simulink model "takeoff_real23B"  (R2023b)
settings: Solver=ode4  StartTime=0.0  StopTime=150  FixedStep=0.001  RelTol=1e-3
values from neighbouring files (symbols this model uses):
  a0 = 340.294    [basedata.m]    (also in basedata.mat; control_design.mat; landing_init.m; landing_plan.mat)
  b_ref = 2.0    (= 2)    [basedata.m]    (also in basedata.mat; control_design.mat; landing_init.m; landing_plan.mat)
  c_gear = [0.8e4, 1.4e4, 1.4e4]    [basedata.m]    (also in basedata.mat = [8000 14000 14000]; control_design.mat = [8000 14000 14000]; landing_init.m; landing_plan.mat = [8000 14000 14000])
  c_lat = [1.4e4, 2.2e4, 2.2e4]    [basedata.m]    (also in basedata.mat = [14000 22000 22000]; control_design.mat = [14000 22000 22000]; landing_init.m; landing_plan.mat = [14000 22000 22000])
  c_ref = 0.9    [basedata.m]    (also in basedata.mat; control_design.mat; landing_init.m; landing_plan.mat)
  c_roll = [0.020, 0.018, 0.018]    [basedata.m]    (also in basedata.mat = [0.02 0.018 0.018]; control_design.mat = [0.02 0.018 0.018]; landing_init.m; landing_plan.mat = [0.02 0.018 0.018])
  CD0 = 0.045    [basedata.m]    (also in basedata.mat; canshujisuan.m; control_design.mat; landing_init.m)
  CL0 = 0.083    [basedata.m]    (also in basedata.mat; control_design.mat; landing_init.m; landing_plan.mat)
  CLa = 3.80    (= 3.8)    [basedata.m]    (also in basedata.mat; canshujisuan.m = 2.5; control_design.mat; landing_init.m)
  Clb = -0.08    [basedata.m]    (also in basedata.mat; control_design.mat; landing_init.m; landing_plan.mat)
  Clda = -0.20    (= -0.2)    [basedata.m]    (also in basedata.mat; control_design.mat; landing_init.m; landing_plan.mat)
  CLde = 0.28    [basedata.m]    (also in basedata.mat; control_design.mat; landing_init.m; landing_plan.mat)
  Clp = -0.70    (= -0.7)    [basedata.m]    (also in basedata.mat; control_design.mat; landing_init.m; landing_plan.mat)
  CLq = 4.50    (= 4.5)    [basedata.m]    (also in basedata.mat; canshujisuan.m = 3; control_design.mat; landing_init.m)
  Clr = 0.08    [basedata.m]    (also in basedata.mat; control_design.mat; landing_init.m; landing_plan.mat)
  Cm0 = 0.060    (= 0.06)    [basedata.m]    (also in basedata.mat; control_design.mat; landing_init.m; landing_plan.mat)
  Cma = -0.80    (= -0.8)    [basedata.m]    (also in basedata.mat; control_design.mat; landing_init.m; landing_plan.mat)
  Cmde = -0.90    (= -0.9)    [basedata.m]    (also in basedata.mat; control_design.mat; landing_init.m; landing_plan.mat)
  Cmq = -18.0    (= -18)    [basedata.m]    (also in basedata.mat; control_design.mat; landing_init.m; landing_plan.mat)
  Cnb = 0.25    [basedata.m]    (also in basedata.mat; control_design.mat; landing_init.m; landing_plan.mat)
  Cndr = -0.15    [basedata.m]    (also in basedata.mat; control_design.mat; landing_init.m; landing_plan.mat)
  Cnp = -0.04    [basedata.m]    (also in basedata.mat; control_design.mat; landing_init.m; landing_plan.mat)
  Cnr = -0.45    [basedata.m]    (also in basedata.mat; control_design.mat; landing_init.m; landing_plan.mat)
  CSb = -0.70    (= -0.7)    [basedata.m]    (also in basedata.mat; control_design.mat; landing_init.m; landing_plan.mat)
  CSdr = 0.18    [basedata.m]    (also in basedata.mat; control_design.mat; landing_init.m; landing_plan.mat)
  CSr = 0.12    [basedata.m]    (also in basedata.mat; control_design.mat; landing_init.m; landing_plan.mat)
  D = 0.5 * rho0 * V^2 * S_ref * CD_current    [canshujisuan.m]
  D0 = 1400    [basedata.m]    (also in basedata.mat; control_design.mat = 800; landing.m; landing_init.m)
  da_max = 25    [basedata.m]    (also in basedata.mat; control_design.mat; landing_init.m; landing_plan.mat)
  da_min = -da_max    (= -25)    [basedata.m]    (also in basedata.mat; control_design.mat; landing_init.m; landing_plan.mat)
  de_max = 25    [basedata.m]    (also in basedata.mat; control_design.mat; landing_init.m; landing_plan.mat)
  de_min = -de_max    (= -25)    [basedata.m]    (also in basedata.mat; control_design.mat; landing_init.m; landing_plan.mat)
  DH = pi / 180    (= 0.0174532925199)    [basedata.m]    (also in basedata.mat; control_design.mat; landing_init.m; landing_plan.mat)
  dr_max = 25    [basedata.m]    (also in basedata.mat; control_design.mat; landing_init.m; landing_plan.mat)
  dr_min = -dr_max    (= -25)    [basedata.m]    (also in basedata.mat; control_design.mat; landing_init.m; landing_plan.mat)
  g = 9.80665    [basedata.m]    (also in basedata.mat; canshujisuan.m; control_design.mat; landing_init.m)
  gamma1 = -0.125844364415    [basedata.mat]    (also in landing_trajectory.m = asin(max(min(gamma1_arg, 1), -1)); landingplan.mat)
  gamma2 = -0.0261780104712    [basedata.mat]    (also in landing_trajectory.m = -0.0261799387799; landingplan.mat = 0.0261780104712)
  ground_z = 0.0    (= 0)    [basedata.m]    (also in basedata.mat; control_design.mat; landing_init.m; landing_plan.mat)
  HD = 180 / pi    (= 57.2957795131)    [basedata.m]    (also in basedata.mat; control_design.mat; landing_init.m; landing_plan.mat)
  I = [ Ixx, -Ixy, -Ixz ... (first row only)    [basedata.m]    (also in basedata.mat = [120  0  0; 0  480  0; 0  0  520]; control_design.mat = [120  0  0; 0  480  0; 0  0  520]; landing_init.m; landing_plan.mat = [120  0  0; 0  480  0; 0  0  520])
  K = 0.12    [basedata.m]    (also in basedata.mat; canshujisuan.m = 0.08; control_design.mat; landing_init.m)
  K_alpha = 7.5375    [basedata.mat]    (also in control_design.m = (((wd_pitch^2)-a24))/(2*kesi_pitch*wd_pitch); control_design.mat; controller.m = 5; landingplan.mat)
  k_gear = [1.0e5, 3.0e5, 3.0e5]    [basedata.m]    (also in basedata.mat = [100000 300000 300000]; control_design.mat = [100000 300000 300000]; landing_init.m; landing_plan.mat = [100000 300000 300000])
  Kn_pitch = -0.120095403309    [basedata.mat]    (also in control_design.m = -(2.2*g*(wd_pitch)^2)/(Tr*(((wd_pitch)^2)-a24)*V_control*a34; control_design.mat; controller.m = (2.2*wd^2*g)/(Tr*(wd^2-a24)*V_test*a34); landingplan.mat)
  Kw_pitch = -0.483749055178    [basedata.mat]    (also in control_design.m = -2*kesi_pitch*wd_pitch/a25; control_design.mat; controller.m = -(2*zeta*wd) / a25; landingplan.mat)
  m = 600.0    (= 600)    [basedata.m]    (also in basedata.mat; canshujisuan.m; control_design.mat; landing_init.m)
  mu_brake = [0.0, 0.55, 0.55]    [basedata.m]    (also in basedata.mat = [0 0.55 0.55]; control_design.mat = [0 0.55 0.55]; landing_init.m; landing_plan.mat = [0 0.55 0.55])
  phi0 = 0    [control_design.mat]    (also in landing.m; landing_init.m; landing_init.mat; landing_plan.mat)
  psi0 = 0    [control_design.mat]    (also in landing.m; landing_init.m; landing_init.mat; landing_plan.mat)
  r_left_b = r_gear_b(:,2)    [basedata.m]    (also in basedata.mat = [-0.333333333333 -0.8 0.65]; control_design.mat = [-0.333333333333 -0.8 0.65]; landing_init.m; landing_plan.mat = [-0.333333333333 -0.8 0.65])
  r_nose_b = r_gear_b(:,1)    [basedata.m]    (also in basedata.mat = [2 0 0.65]; control_design.mat = [2 0 0.65]; landing_init.m; landing_plan.mat = [2 0 0.65])
  r_right_b = r_gear_b(:,3)    [basedata.m]    (also in basedata.mat = [-0.333333333333 0.8 0.65]; control_design.mat = [-0.333333333333 0.8 0.65]; landing_init.m; landing_plan.mat = [-0.333333333333 0.8 0.65])
  rho0 = 1.225    [basedata.m]    (also in basedata.mat; canshujisuan.m; control_design.mat; landing_init.m)
  S_ref = 1.2    [basedata.m]    (also in basedata.mat; canshujisuan.m; control_design.mat; landing_init.m)
  theta0 = 0    [control_design.mat]    (also in landing.m; landing_init.m; landing_init.mat = 0.0523598775598; landing_plan.mat = 0.0523560209424)
  u0_b = 0    [control_design.mat]    (also in landing.m = 128; landing_init.m = 128; landing_init.mat = 100; landing_plan.mat = 128)
  v0_b = 0    [control_design.mat]    (also in landing.m; landing_init.m; landing_init.mat; landing_plan.mat)
  V_app = 128.516392565    [basedata.mat]    (also in landing_trajectory.m = 1.4 * Vs; landingplan.mat)
  v_eps = 0.20    (= 0.2)    [basedata.m]    (also in basedata.mat; control_design.mat; landing_init.m; landing_plan.mat)
  V_flare = V_shallow    [landing_trajectory.m]
  V_min = 3    [control_design.mat]    (also in landing.m; landing_init.m; landing_plan.mat; landingplan.mat)
  V_shallow = 110.156907913    [basedata.mat]    (also in landing_trajectory.m = 1.2 * Vs; landingplan.mat)
  w0_b = 0    [control_design.mat]    (also in landing.m; landing_init.m; landing_init.mat; landing_plan.mat)
  wheel_radius = 0.18    [basedata.m]    (also in basedata.mat; control_design.mat; landing_init.m; landing_plan.mat)
  WOW_on = 0.000    (= 0)    [basedata.m]    (also in basedata.mat; control_design.mat; landing_init.m; landing_plan.mat)
  X_B = -4048.29417932    [basedata.mat]    (also in landing_trajectory.m = X_R - R * sin(a1); landingplan.mat)
  X_C = -3253.59462264    [basedata.mat]    (also in landing_trajectory.m = X_R - R * sin(a2); landingplan.mat)
  X_D = -1263.82547196    [basedata.mat]    (also in landing_trajectory.m = X_aim - H_exp / tan(a2); landingplan.mat)
  X_entry = -10904.3307826    [basedata.mat]    (also in landing_trajectory.m = X_zero - H_entry / tan(a1); landingplan.mat)
  Xg0 = 0    [control_design.mat]    (also in landing.m = -12000; landing_init.m = -12000; landing_init.mat = -8000; landing_plan.mat = -12000)
  Yg0 = 3    [control_design.mat]    (also in landing.m = 0; landing_init.m = 0; landing_init.mat = 0; landing_plan.mat = 0)
  Zg0 = ground_z - wheel_radius - r_gear_b(3,1) + static_deflection    [basedata.m]    (also in basedata.mat = -0.8215943; control_design.mat = -0.8215943; landing.m = -1000; landing_init.m = -1000)
undefined symbols (not defined in the file or in its folder): I_xz, I_yz, Ix_Iy, Iy_Iz, Iz_Ix
libraries: simulink x64, matrix_library x19
(part 1 of 4)
settings Model: Creator=34355  LastModifiedBy=fjy
settings DataIOCC: SaveFormat=StructureWithTime  SaveState=on  SignalLogging=off
settings RTWCC: GPUComputeCapability=5.0
settings ConfigComp: CovBoundaryAbsTol=1.0e-5

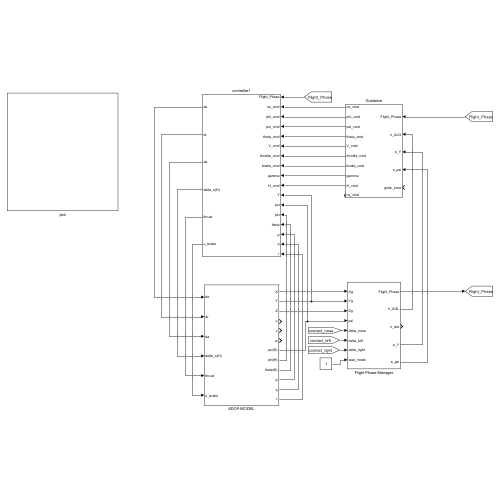
[thumbnail: Simulink's stored preview of the top-level diagram]
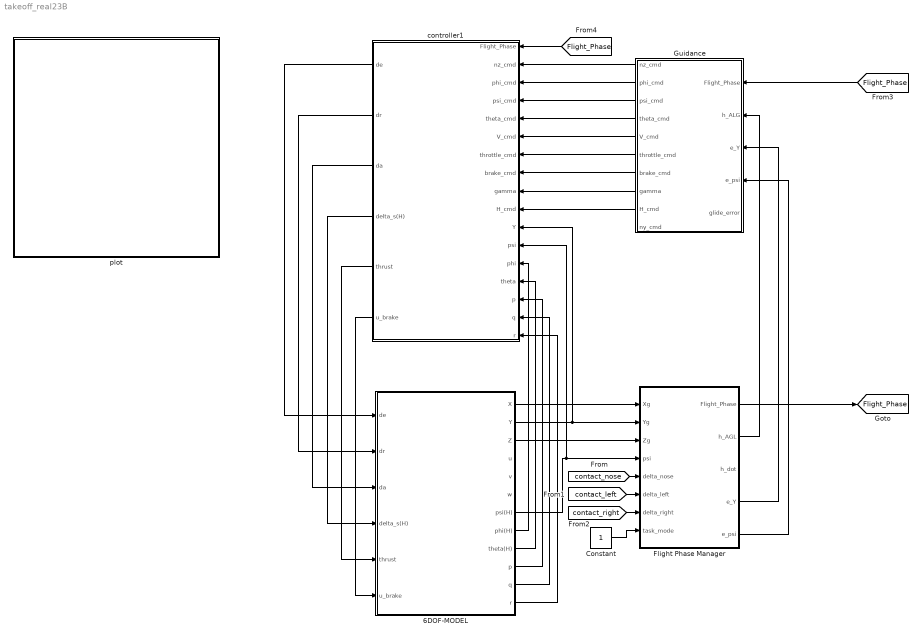
== system takeoff_real23B ==
  6DOF-MODEL : Subsystem
  Constant : Constant
  Flight Phase Manager : Subsystem
  Guidance : Subsystem
  controller1 : Subsystem
  plot : Subsystem
  tag scope: Flight_Phase=global
  wires:
  Constant/1 -> Flight Phase Manager/8(task_mode)
  6DOF-MODEL/1(X) -> Flight Phase Manager/1(Xg)
  6DOF-MODEL/2(Y) -> Flight Phase Manager/2(Yg), controller1/11(Y)
  6DOF-MODEL/3(Z) -> Flight Phase Manager/3(Zg)
  6DOF-MODEL/7(psi(H)) -> controller1/12(psi), Flight Phase Manager/4(psi)
  [contact_nose] -> Flight Phase Manager/5(delta_nose)
  [contact_left] -> Flight Phase Manager/6(delta_left)
  [contact_right] -> Flight Phase Manager/7(delta_right)
  Flight Phase Manager/1(Flight_Phase) -> [Flight_Phase]
  Flight Phase Manager/2(h_AGL) -> Guidance/2(h_ALG)
  Flight Phase Manager/4(e_Y) -> Guidance/3(e_Y)
  Flight Phase Manager/5(e_psi) -> Guidance/4(e_psi)
  Guidance/1(nz_cmd) -> controller1/2(nz_cmd)
  Guidance/2(phi_cmd) -> controller1/3(phi_cmd)
  Guidance/3(psi_cmd) -> controller1/4(psi_cmd)
  Guidance/4(theta_cmd) -> controller1/5(theta_cmd)
  Guidance/5(V_cmd) -> controller1/6(V_cmd)
  Guidance/6(throttle_cmd) -> controller1/7(throttle_cmd)
  Guidance/7(brake_cmd) -> controller1/8(brake_cmd)
  6DOF-MODEL/8(phi(H)) -> controller1/13(phi)
  6DOF-MODEL/9(theta(H)) -> controller1/14(theta)
  6DOF-MODEL/10(p) -> controller1/15(p)
  6DOF-MODEL/11(q) -> controller1/16(q)
  6DOF-MODEL/12(r) -> controller1/17(r)
  controller1/1(de) -> 6DOF-MODEL/1(de)
  controller1/2(dr) -> 6DOF-MODEL/2(dr)
  controller1/3(da) -> 6DOF-MODEL/3(da)
  controller1/4(delta_s(H)) -> 6DOF-MODEL/4(delta_s(H))
  controller1/5(thrust) -> 6DOF-MODEL/5(thrust)
  controller1/6(u_brake) -> 6DOF-MODEL/6(u_brake)
  Guidance/8(gamma) -> controller1/9(gamma)
  Guidance/9(H_cmd) -> controller1/10(H_cmd)
  [Flight_Phase] -> Guidance/1(Flight_Phase)
  [Flight_Phase] -> controller1/1(Flight_Phase)

== system takeoff_real23B/6DOF-MODEL ==
  de : Inport
  dr : Inport  Port=2
  da : Inport  Port=3
  delta_s(H) : Inport  Port=4
  thrust : Inport  Port=5
  u_brake : Inport  Port=6
  AERO-PARAMETER : Subsystem
  Scope : Scope
  Scope5 : Scope
  Scope6 : Scope
  动力学 : Subsystem
  X : Outport
  Y : Outport  Port=2
  Z : Outport  Port=3
  u : Outport  Port=4
  v : Outport  Port=5
  w : Outport  Port=6
  psi(H) : Outport  Port=7
  phi(H) : Outport  Port=8
  theta(H) : Outport  Port=9
  p : Outport  Port=10
  q : Outport  Port=11
  r : Outport  Port=12
  wires:
  动力学/1(alpha(D)) -> Scope/1, AERO-PARAMETER/1(alpha(D))
  thrust/1 -> 动力学/7(thrust)
  u_brake/1 -> 动力学/9(u_brake)
  AERO-PARAMETER/1(D) -> Scope6/1, 动力学/1(D)
  AERO-PARAMETER/2(L) -> Scope5/1, 动力学/2(L)
  AERO-PARAMETER/3(S) -> 动力学/3(S)
  AERO-PARAMETER/4(MX) -> 动力学/4(MX)
  AERO-PARAMETER/5(MY) -> 动力学/5(MY)
  AERO-PARAMETER/6(MZ) -> 动力学/6(MZ)
  delta_s(H)/1 -> 动力学/8(delta_s(H))
  动力学/2(beta(D)) -> AERO-PARAMETER/2(beta(D))
  动力学/3(p) -> p/1, AERO-PARAMETER/3(p(H))
  动力学/4(q) -> q/1, AERO-PARAMETER/4(q(H))
  动力学/5(r) -> r/1, AERO-PARAMETER/5(r(H))
  de/1 -> AERO-PARAMETER/6(de(D))
  dr/1 -> AERO-PARAMETER/7(dr(D))
  da/1 -> AERO-PARAMETER/8(da)
  动力学/14(w) -> w/1
  动力学/7(Y) -> Y/1
  动力学/8(Z) -> Z/1
  动力学/13(v) -> v/1
  动力学/11(psi(H)) -> psi(H)/1
  动力学/12(u) -> u/1
  动力学/10(theta(H)) -> theta(H)/1
  动力学/6(X) -> X/1
  动力学/9(phi(H)) -> phi(H)/1

== system takeoff_real23B/Flight Phase Manager ==
  Xg : Inport
  Yg : Inport  Port=2
  Zg : Inport  Port=3
  psi : Inport  Port=4
  delta_nose : Inport  Port=5
  delta_left : Inport  Port=6
  delta_right : Inport  Port=7
  task_mode : Inport  Port=8
  Data Pre-processing : Subsystem
  Phase Logic : Stateflow chart  TreatAsAtomicUnit=on
      settings: PortSchema="{\"entries\":[{\"content\":{\"sides\":[{\"content\":{\"connectorIds\":[\"In1\",\"In2\",\"In3\",\"In4\",\"In5\",\"In6\",\"In7\",\"In8\",\"In9\",\"In10\",\"In11\",\"In14\",\"In16\",\"In15\",\"In12\",\"In13\"]},\"type\":\"ConnectorPlacement.EquallySpacedRectSide\",\"uuid\":\"d1377902-4c9e-4853-af6d-27f5bb7637ce\"},{\"content\":{\"connectorIds\":[\"Out1\"],\"side\":\"RIGHT\"},\"type\":\"ConnectorPlacement.EquallySpacedRectSide\",\"uuid\":\"199ad0df-8e84-4c58-a318-47ec4e7019a7\"},{\"content\":{\"side\":\"TOP\"},\"type\":\"ConnectorPlacement.EquallySpacedRectSide\",\"uuid\":\"128f90a0-f282-43f5-aaeb-01018f5264b1\"}]},\"type\":\"ConnectorPlacement.EquallySpacedConnector\",\"uuid\":\"57900c2f-d5fa-4b9f-a9e2-0e52881776fd\"}],\"packageUris\":[\"http://schema.mathworks.com/mf0/Connector/R2020b\"],\"version\":\"1.0\"}"
  Flight_Phase : Outport
  h_AGL : Outport  Port=2
  h_dot : Outport  Port=3
  e_Y : Outport  Port=4
  e_psi : Outport  Port=5
  wires:
  Xg/1 -> Data Pre-processing/1(Xg)
  Yg/1 -> Data Pre-processing/2(Yg)
  Zg/1 -> Data Pre-processing/3(Zg)
  psi/1 -> Data Pre-processing/4(psi)
  delta_nose/1 -> Data Pre-processing/5(delta_nose)
  delta_left/1 -> Data Pre-processing/6(delta_left)
  delta_right/1 -> Data Pre-processing/7(delta_right)
  Phase Logic/1(Flight_Phase) -> Flight_Phase/1
  task_mode/1 -> Phase Logic/13(Task_Mode)
  Data Pre-processing/1(h_AGL) -> Phase Logic/1(h_AGL), h_AGL/1
  Data Pre-processing/2(V_runway) -> Phase Logic/2(V_runway)
  Data Pre-processing/3(h_dot) -> Phase Logic/3(h_dot), h_dot/1
  Data Pre-processing/4(nose_on_ground) -> Phase Logic/4(nose_on_ground)
  Data Pre-processing/5(main_on_ground) -> Phase Logic/5(main_on_ground)
  Data Pre-processing/6(airborne) -> Phase Logic/6(airborne)
  Data Pre-processing/7(reach_VR) -> Phase Logic/7(reach_VR)
  Data Pre-processing/8(safe_climb) -> Phase Logic/8(safe_climb)
  Data Pre-processing/9(localizer_captured) -> Phase Logic/9(localizer_captured)
  Data Pre-processing/10(glideslope_captured) -> Phase Logic/10(glideslope_captured)
  Data Pre-processing/11(flare_entry) -> Phase Logic/11(flare_entry)
  Data Pre-processing/15(stop_condition) -> Phase Logic/12(stop_condition)
  Data Pre-processing/17(e_Y) -> e_Y/1
  Data Pre-processing/16(e_psi) -> e_psi/1
  Data Pre-processing/12(In_round) -> Phase Logic/14(in_round)
  Data Pre-processing/13(Slight decline) -> Phase Logic/16(Slight_decline)
  Data Pre-processing/14(in_flare) -> Phase Logic/15(in_Flare)

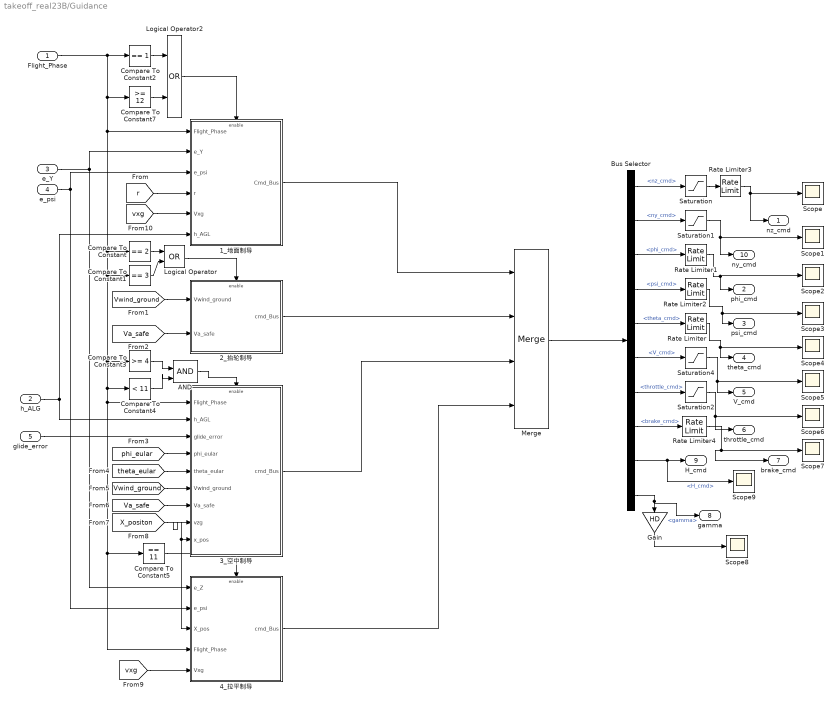
== system takeoff_real23B/Guidance ==
  Flight_Phase : Inport
  h_ALG : Inport  Port=2
  e_Y : Inport  Port=3
  e_psi : Inport  Port=4
  glide_error : Inport  Port=5
  1_地面制导 : Subsystem
  "2_抬轮制导 " : Subsystem
  3_空中制导 : Subsystem
  4_拉平制导 : Subsystem
  AND : Logic  IconShape=distinctive  AllPortsSameDT=off  OutDataTypeStr=boolean
  Bus Selector : BusSelector  OutputSignals=nz_cmd,ny_cmd,phi_cmd,psi_cmd,theta_cmd,V_cmd,throttle_cmd,brake_cmd,H_cmd,gamma
  Compare To Constant : simulink/Logic and Bit Operations/Compare To Constant  relop===  const=2  OutDataTypeStr=boolean
  Compare To Constant1 : simulink/Logic and Bit Operations/Compare To Constant  relop===  const=3  OutDataTypeStr=boolean
  Compare To Constant2 : simulink/Logic and Bit Operations/Compare To Constant  relop===  const=1  OutDataTypeStr=boolean
  Compare To Constant3 : simulink/Logic and Bit Operations/Compare To Constant  relop=>=  const=4  OutDataTypeStr=boolean
  Compare To Constant4 : simulink/Logic and Bit Operations/Compare To Constant  relop=<  const=11  OutDataTypeStr=boolean
  Compare To Constant5 : simulink/Logic and Bit Operations/Compare To Constant  relop===  const=11  OutDataTypeStr=boolean
  Compare To Constant7 : simulink/Logic and Bit Operations/Compare To Constant  relop=>=  const=12  OutDataTypeStr=boolean
  Gain : Gain  Gain=HD
  Logical Operator : Logic  Operator=OR  AllPortsSameDT=off  OutDataTypeStr=boolean
  Logical Operator2 : Logic  Operator=OR  AllPortsSameDT=off  OutDataTypeStr=boolean
  Merge : Merge  Inputs=4
  Rate Limiter : RateLimiter  RisingSlewLimit=1*DH  FallingSlewLimit=-1*DH  SampleTimeMode=inherited
  Rate Limiter1 : RateLimiter  RisingSlewLimit=10*DH  FallingSlewLimit=-10*DH  SampleTimeMode=inherited
  Rate Limiter2 : RateLimiter  RisingSlewLimit=10*DH  FallingSlewLimit=-10*DH  SampleTimeMode=inherited
  Rate Limiter3 : RateLimiter  RisingSlewLimit=0.8  FallingSlewLimit=-0.8  SampleTimeMode=inherited
  Rate Limiter4 : RateLimiter  RisingSlewLimit=0.2  FallingSlewLimit=-0.2  SampleTimeMode=inherited
  Saturation : Saturate  UpperLimit=2  LowerLimit=-2
  Saturation1 : Saturate  UpperLimit=2  LowerLimit=-2
  Saturation2 : Saturate  UpperLimit=1  LowerLimit=0
  Saturation4 : Saturate  UpperLimit=250  LowerLimit=0
  Scope{,1..9} (10 alike) : Scope
  nz_cmd : Outport
  phi_cmd : Outport  Port=2
  psi_cmd : Outport  Port=3
  theta_cmd : Outport  Port=4
  V_cmd : Outport  Port=5
  throttle_cmd : Outport  Port=6
  brake_cmd : Outport  Port=7
  gamma : Outport  Port=8
  H_cmd : Outport  Port=9
  ny_cmd : Outport  Port=10
  wires:
  Flight_Phase/1 -> Compare To Constant4/1, 4_拉平制导/4(Flight_Phase), Compare To Constant5/1, 3_空中制导/1(Flight_Phase), Compare To Constant3/1, Compare To Constant1/1, Compare To Constant/1, 1_地面制导/1(Flight_Phase), Compare To Constant7/1, Compare To Constant2/1
  e_Y/1 -> 4_拉平制导/1(e_Z), 1_地面制导/2(e_Y)
  Merge/1 -> Bus Selector/1
  e_psi/1 -> 4_拉平制导/2(e_psi), 1_地面制导/3(e_psi)
  h_ALG/1 -> 3_空中制导/2(h_AGL), 1_地面制导/6(h_AGL)
  glide_error/1 -> 3_空中制导/3(glide_error)
  Saturation1/1 -> ny_cmd/1, Scope1/1
  Compare To Constant/1 -> Logical Operator/1
  Compare To Constant1/1 -> Logical Operator/2
  Logical Operator/1 -> "2_抬轮制导 "/Enable
  Compare To Constant5/1 -> 4_拉平制导/Enable
  Compare To Constant2/1 -> Logical Operator2/1
  Logical Operator2/1 -> 1_地面制导/Enable
  Rate Limiter/1 -> theta_cmd/1, Scope4/1
  Rate Limiter1/1 -> phi_cmd/1, Scope2/1
  3_空中制导/1(cmd_Bus) -> Merge/3
  Rate Limiter2/1 -> psi_cmd/1, Scope3/1
  Rate Limiter4/1 -> brake_cmd/1, Scope7/1
  Saturation4/1 -> V_cmd/1, Scope5/1
  Saturation/1 -> Rate Limiter3/1
  Rate Limiter3/1 -> nz_cmd/1, Scope/1
  Saturation2/1 -> throttle_cmd/1, Scope6/1
  [r] -> 1_地面制导/4(r)
  [Vwind_ground] -> "2_抬轮制导 "/1(Vwind_ground)
  [Va_safe] -> "2_抬轮制导 "/2(Va_safe)
  [phi_eular] -> 3_空中制导/4(phi_eular)
  [theta_eular] -> 3_空中制导/5(theta_eular)
  [Vwind_ground] -> 3_空中制导/6(Vwind_ground)
  [Va_safe] -> 3_空中制导/7(Va_safe)
  Bus Selector/1 -> Saturation/1  "<nz_cmd>"
  Bus Selector/2 -> Saturation1/1  "<ny_cmd>"
  Bus Selector/3 -> Rate Limiter1/1  "<phi_cmd>"
  Bus Selector/4 -> Rate Limiter2/1  "<psi_cmd>"
  Bus Selector/5 -> Rate Limiter/1  "<theta_cmd>"
  Bus Selector/6 -> Saturation4/1  "<V_cmd>"
  Bus Selector/7 -> Saturation2/1  "<throttle_cmd>"
  Bus Selector/8 -> Rate Limiter4/1  "<brake_cmd>"
  [vzg] -> 3_空中制导/8(vzg)
  [X_positon] -> 4_拉平制导/3(X_pos), 3_空中制导/9(x_pos)
  Bus Selector/10 -> gamma/1, Gain/1  "<gamma>"
  Bus Selector/9 -> Scope9/1, H_cmd/1  "<H_cmd>"
  Gain/1 -> Scope8/1
  1_地面制导/1(Cmd_Bus) -> Merge/1
  "2_抬轮制导 "/1(cmd_Bus) -> Merge/2
  4_拉平制导/1(cmd_Bus) -> Merge/4
  Compare To Constant7/1 -> Logical Operator2/2
  [vxg] -> 4_拉平制导/5(Vxg)
  [vxg] -> 1_地面制导/5(Vxg)
  Compare To Constant3/1 -> AND/1
  Compare To Constant4/1 -> AND/2
  AND/1 -> 3_空中制导/Enable

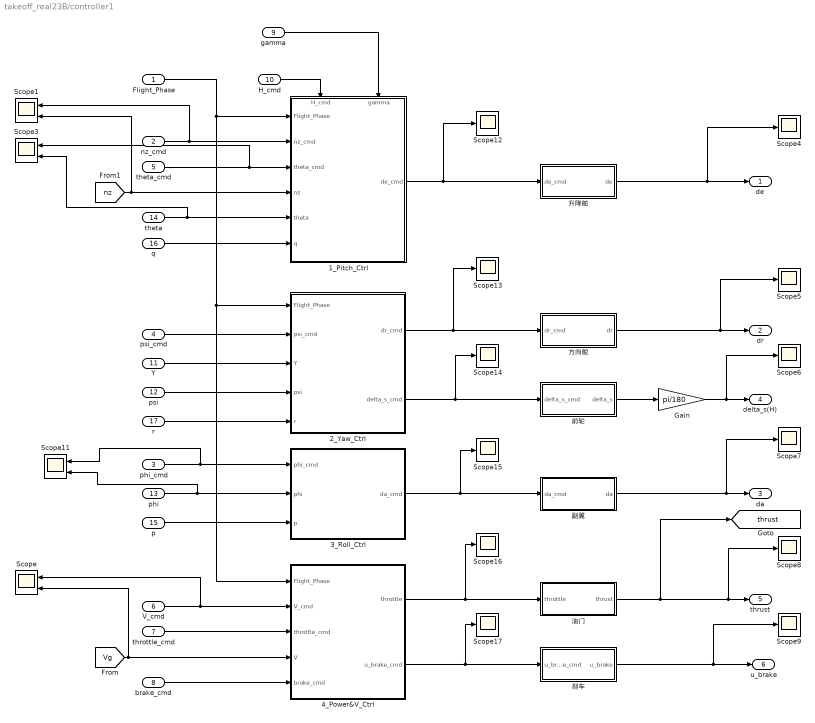
== system takeoff_real23B/controller1 ==
  Flight_Phase : Inport
  nz_cmd : Inport  Port=2
  phi_cmd : Inport  Port=3
  psi_cmd : Inport  Port=4
  theta_cmd : Inport  Port=5
  V_cmd : Inport  Port=6
  throttle_cmd : Inport  Port=7
  brake_cmd : Inport  Port=8
  gamma : Inport  Port=9
  H_cmd : Inport  Port=10
  Y : Inport  Port=11
  psi : Inport  Port=12
  phi : Inport  Port=13
  theta : Inport  Port=14
  p : Inport  Port=15
  q : Inport  Port=16
  r : Inport  Port=17
  1_Pitch_Ctrl : Subsystem
      settings: PortSchema="{\"entries\":[{\"content\":{\"sides\":[{\"content\":{\"connectorIds\":[\"In1\",\"In2\",\"In3\",\"In4\",\"In5\",\"In6\"]},\"type\":\"ConnectorPlacement.EquallySpacedRectSide\",\"uuid\":\"27d13232-9f89-4ac1-9c77-5758657de7c7\"},{\"content\":{\"connectorIds\":[\"Out1\"],\"side\":\"RIGHT\"},\"type\":\"ConnectorPlacement.EquallySpacedRectSide\",\"uuid\":\"ae62ad8c-a405-4422-b5ec-9ac723f70591\"},{\"content\":{\"connectorIds\":[\"In7\",\"In8\"],\"side\":\"TOP\"},\"type\":\"ConnectorPlacement.EquallySpacedRectSide\",\"uuid\":\"4cebe0f4-d768-4fb6-931c-2fd4183255b7\"}]},\"type\":\"ConnectorPlacement.EquallySpacedConnector\",\"uuid\":\"2c44e0df-7f94-4dab-9232-216c905b911f\"}],\"packageUris\":[\"http://schema.mathworks.com/mf0/Connector/R2020b\"],\"version\":\"1.0\"}"
  2_Yaw_Ctrl : Subsystem
  3_Roll_Ctrl : Subsystem
  4_Power&V_Ctrl : Subsystem
  Gain : Gain  Gain=pi/180
  Scope{,1,3,11} (4 alike) : Scope  NumInputPorts=2
  Scope{4..9,12..17} (12 alike) : Scope
  刹车 : Subsystem
  前轮 : Subsystem
  副翼 : Subsystem
  升降舵 : Subsystem
  方向舵 : Subsystem
  油门 : Subsystem
  de : Outport
  dr : Outport  Port=2
  da : Outport  Port=3
  delta_s(H) : Outport  Port=4
  thrust : Outport  Port=5
  u_brake : Outport  Port=6
  tag scope: thrust=global
  wires:
  phi_cmd/1 -> Scope11/1, 3_Roll_Ctrl/1(phi_cmd)
  phi/1 -> Scope11/2, 3_Roll_Ctrl/2(phi)
  p/1 -> 3_Roll_Ctrl/3(p)
  brake_cmd/1 -> 4_Power&V_Ctrl/5(brake_cmd)
  4_Power&V_Ctrl/1(throttle) -> 油门/1(throttle), Scope16/1
  Flight_Phase/1 -> 1_Pitch_Ctrl/1(Flight_Phase), 2_Yaw_Ctrl/1(Flight_Phase), 4_Power&V_Ctrl/1(Flight_Phase)
  nz_cmd/1 -> Scope1/1, 1_Pitch_Ctrl/2(nz_cmd)
  psi_cmd/1 -> 2_Yaw_Ctrl/2(psi_cmd)
  [nz] -> Scope1/2, 1_Pitch_Ctrl/4(nz)
  q/1 -> 1_Pitch_Ctrl/6(q)
  V_cmd/1 -> Scope/1, 4_Power&V_Ctrl/2(V_cmd)
  [Vg] -> Scope/2, 4_Power&V_Ctrl/4(V)
  Gain/1 -> Scope6/1, delta_s(H)/1
  theta_cmd/1 -> Scope3/1, 1_Pitch_Ctrl/3(theta_cmd)
  1_Pitch_Ctrl/1(de_cmd) -> 升降舵/1(de_cmd), Scope12/1
  2_Yaw_Ctrl/1(dr_cmd) -> Scope13/1, 方向舵/1(dr_cmd)
  2_Yaw_Ctrl/2(delta_s_cmd) -> Scope14/1, 前轮/1(delta_s_cmd)
  3_Roll_Ctrl/1(da_cmd) -> Scope15/1, 副翼/1(da_cmd)
  4_Power&V_Ctrl/2(u_brake_cmd) -> 刹车/1(u_brake_cmd), Scope17/1
  theta/1 -> Scope3/2, 1_Pitch_Ctrl/5(theta)
  throttle_cmd/1 -> 4_Power&V_Ctrl/3(throttle_cmd)
  Y/1 -> 2_Yaw_Ctrl/3(Y)
  psi/1 -> 2_Yaw_Ctrl/4(psi)
  r/1 -> 2_Yaw_Ctrl/5(r)
  升降舵/1(de) -> Scope4/1, de/1
  方向舵/1(dr) -> Scope5/1, dr/1
  前轮/1(delta_s) -> Gain/1
  副翼/1(da) -> Scope7/1, da/1
  油门/1(thrust) -> [thrust], Scope8/1, thrust/1
  刹车/1(u_brake) -> Scope9/1, u_brake/1
  H_cmd/1 -> 1_Pitch_Ctrl/7(H_cmd)
  gamma/1 -> 1_Pitch_Ctrl/8(gamma)

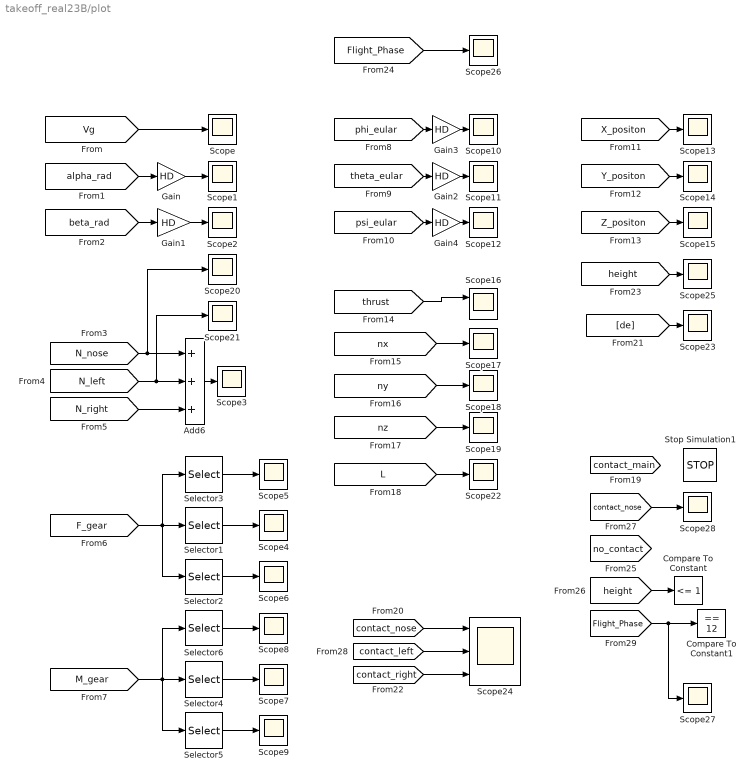
== system takeoff_real23B/plot ==
  Add6 : Sum  Inputs=+++
  Compare To Constant : simulink/Logic and Bit Operations/Compare To Constant  relop=<=  const=1  OutDataTypeStr=boolean
  Compare To Constant1 : simulink/Logic and Bit Operations/Compare To Constant  relop===  const=12  OutDataTypeStr=boolean
  Gain{,1..4} (5 alike) : Gain  Gain=HD
  Scope{,1..15,17..23,25..28} (27 alike) : Scope
  Scope16 : Scope  NumInputPorts=2
  Scope24 : Scope  NumInputPorts=3
  Selector1 : Selector  InputPortWidth=3  IndexOptions=Index vector (dialog)  Indices=2  OutputSizes=1
  Selector2 : Selector  InputPortWidth=3  IndexOptions=Index vector (dialog)  Indices=3  OutputSizes=1
  Selector3 : Selector  InputPortWidth=3  IndexOptions=Index vector (dialog)  Indices=1  OutputSizes=1
  Selector4 : Selector  InputPortWidth=3  IndexOptions=Index vector (dialog)  Indices=2  OutputSizes=1
  Selector5 : Selector  InputPortWidth=3  IndexOptions=Index vector (dialog)  Indices=3  OutputSizes=1
  Selector6 : Selector  InputPortWidth=3  IndexOptions=Index vector (dialog)  Indices=1  OutputSizes=1
  Stop Simulation1 : Stop
  wires:
  [N_nose] -> Add6/1, Scope20/1
  [N_left] -> Scope21/1, Add6/2
  [N_right] -> Add6/3
  [Vg] -> Scope/1
  [alpha_rad] -> Gain/1
  [beta_rad] -> Gain1/1
  Add6/1 -> Scope3/1
  Selector3/1 -> Scope5/1
  Selector2/1 -> Scope6/1
  Selector1/1 -> Scope4/1
  [F_gear] -> Selector2/1, Selector1/1, Selector3/1
  Selector6/1 -> Scope8/1
  Selector4/1 -> Scope7/1
  [M_gear] -> Selector6/1, Selector4/1, Selector5/1
  Selector5/1 -> Scope9/1
  [psi_eular] -> Gain4/1
  [theta_eular] -> Gain2/1
  [phi_eular] -> Gain3/1
  Gain1/1 -> Scope2/1
  Gain/1 -> Scope1/1
  Gain2/1 -> Scope11/1
  [Y_positon] -> Scope14/1
  [X_positon] -> Scope13/1
  [Z_positon] -> Scope15/1
  Gain3/1 -> Scope10/1
  Gain4/1 -> Scope12/1
  [thrust] -> Scope16/1
  [nx] -> Scope17/1
  [ny] -> Scope18/1
  [nz] -> Scope19/1
  [L] -> Scope22/1
  [de] -> Scope23/1
  [height] -> Scope25/1
  [height] -> Compare To Constant/1
  [contact_left] -> Scope24/2
  [contact_right] -> Scope24/3
  [Flight_Phase] -> Scope26/1
  [Flight_Phase] -> Compare To Constant1/1, Scope27/1
  [contact_nose] -> Scope28/1
  [contact_nose] -> Scope24/1

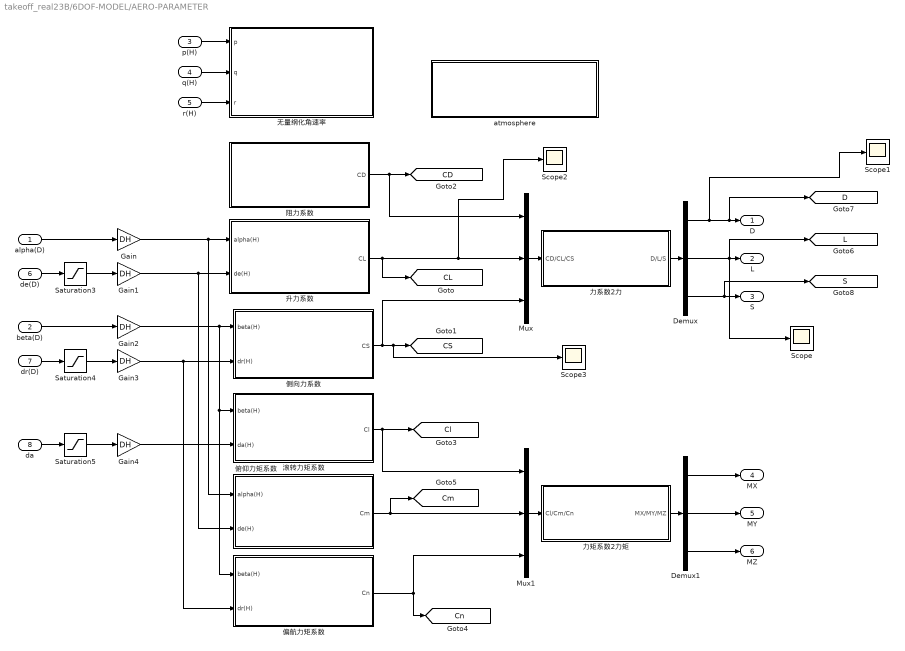
== system takeoff_real23B/6DOF-MODEL/AERO-PARAMETER ==
  alpha(D) : Inport
  beta(D) : Inport  Port=2
  p(H) : Inport  Port=3
  q(H) : Inport  Port=4
  r(H) : Inport  Port=5
  de(D) : Inport  Port=6
  dr(D) : Inport  Port=7
  da : Inport  Port=8
  Demux : Demux  Outputs=3
  Demux1 : Demux  Outputs=3
  Gain{,1..4} (5 alike) : Gain  Gain=DH
  Mux : Mux  Inputs=3
  Mux1 : Mux  Inputs=3
  Saturation3 : Saturate  UpperLimit=de_max  LowerLimit=de_min
  Saturation4 : Saturate  UpperLimit=dr_max  LowerLimit=dr_min
  Saturation5 : Saturate  UpperLimit=da_max  LowerLimit=da_min
  Scope{,1..3} (4 alike) : Scope
  atmosphere : Subsystem
  侧向力系数 : Subsystem
  俯仰力矩系数 : Subsystem
  偏航力矩系数 : Subsystem
  力矩系数2力矩 : Subsystem
  力系数2力 : Subsystem
  升力系数 : Subsystem
  无量纲化角速率 : Subsystem
  滚转力矩系数 : Subsystem
  阻力系数 : Subsystem
  D : Outport
  L : Outport  Port=2
  S : Outport  Port=3
  MX : Outport  Port=4
  MY : Outport  Port=5
  MZ : Outport  Port=6
  tag scope: CD=global, CL=global, CS=global, Cl=global, Cm=global, Cn=global, D=global, L=global, S=global
  wires:
  升力系数/1(CL) -> [CL], Scope2/1, Mux/2
  侧向力系数/1(CS) -> Mux/3, Scope3/1, [CS]
  da/1 -> Saturation5/1
  Saturation5/1 -> Gain4/1
  Saturation4/1 -> Gain3/1
  dr(D)/1 -> Saturation4/1
  de(D)/1 -> Saturation3/1
  Saturation3/1 -> Gain1/1
  beta(D)/1 -> Gain2/1
  alpha(D)/1 -> Gain/1
  Gain/1 -> 升力系数/1(alpha(H)), 俯仰力矩系数/1(alpha(H))
  Gain1/1 -> 升力系数/2(de(H)), 俯仰力矩系数/2(de(H))
  Gain2/1 -> 侧向力系数/1(beta(H)), 偏航力矩系数/1(beta(H)), 滚转力矩系数/1(beta(H))
  Gain3/1 -> 侧向力系数/2(dr(H)), 偏航力矩系数/2(dr(H))
  Gain4/1 -> 滚转力矩系数/2(da(H))
  p(H)/1 -> 无量纲化角速率/1(p)
  q(H)/1 -> 无量纲化角速率/2(q)
  r(H)/1 -> 无量纲化角速率/3(r)
  阻力系数/1(CD) -> Mux/1, [CD]
  滚转力矩系数/1(Cl) -> [Cl], Mux1/1
  俯仰力矩系数/1(Cm) -> Mux1/2, [Cm]
  偏航力矩系数/1(Cn) -> [Cn], Mux1/3
  Mux/1 -> 力系数2力/1(CD/CL/CS)
  Mux1/1 -> 力矩系数2力矩/1(Cl/Cm/Cn)
  Demux/2 -> Scope/1, [L], L/1
  力系数2力/1(D/L/S) -> Demux/1
  Demux/1 -> Scope1/1, [D], D/1
  Demux/3 -> [S], S/1
  力矩系数2力矩/1(MX/MY/MZ) -> Demux1/1
  Demux1/1 -> MX/1
  Demux1/2 -> MY/1
  Demux1/3 -> MZ/1

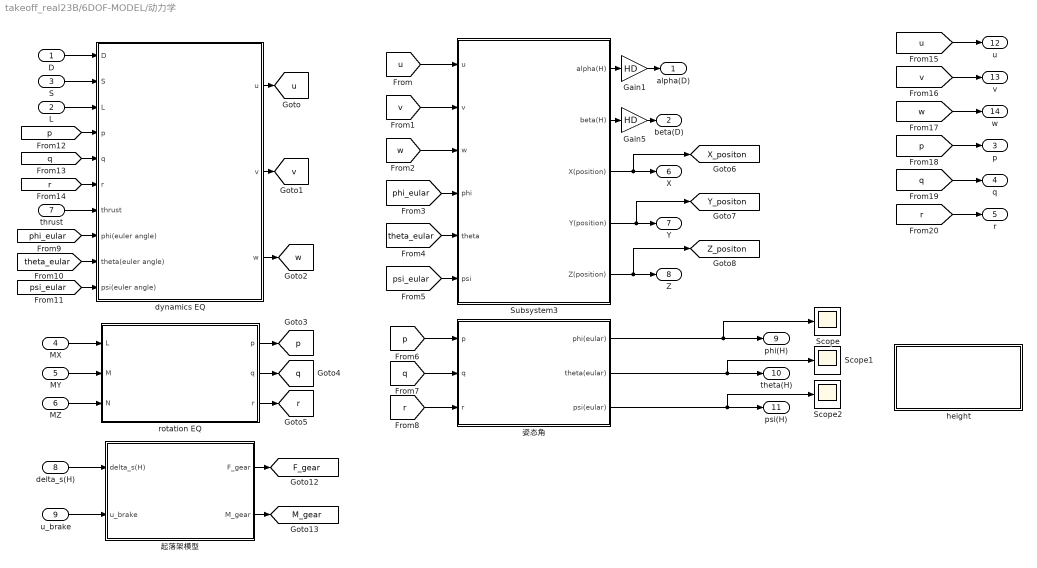
== system takeoff_real23B/6DOF-MODEL/动力学 ==
  D : Inport
  L : Inport  Port=2
  S : Inport  Port=3
  MX : Inport  Port=4
  MY : Inport  Port=5
  MZ : Inport  Port=6
  thrust : Inport  Port=7
  delta_s(H) : Inport  Port=8
  u_brake : Inport  Port=9
  Gain1 : Gain  Gain=HD
  Gain5 : Gain  Gain=HD
  Scope : Scope
  Scope1 : Scope
  Scope2 : Scope
  Subsystem3 : Subsystem
  dynamics EQ : Subsystem
  height : Subsystem
  rotation EQ : Subsystem
  姿态角 : Subsystem
  起落架模型 : Subsystem
  alpha(D) : Outport
  beta(D) : Outport  Port=2
  p : Outport  Port=3
  q : Outport  Port=4
  r : Outport  Port=5
  X : Outport  Port=6
  Y : Outport  Port=7
  Z : Outport  Port=8
  phi(H) : Outport  Port=9
  theta(H) : Outport  Port=10
  psi(H) : Outport  Port=11
  u : Outport  Port=12
  v : Outport  Port=13
  w : Outport  Port=14
  tag scope: F_gear=global, M_gear=global, X_positon=global, Y_positon=global, Z_positon=global, p=global, q=global, r=global, u=global, v=global, w=global
  wires:
  姿态角/1(phi(eular)) -> Scope/1, phi(H)/1
  姿态角/2(theta(eular)) -> theta(H)/1, Scope1/1
  姿态角/3(psi(eular)) -> psi(H)/1, Scope2/1
  Gain5/1 -> beta(D)/1
  Gain1/1 -> alpha(D)/1
  [u] -> u/1
  [v] -> v/1
  [w] -> w/1
  [p] -> p/1
  [q] -> q/1
  [r] -> r/1
  起落架模型/1(F_gear) -> [F_gear]
  起落架模型/2(M_gear) -> [M_gear]
  MX/1 -> rotation EQ/1(L)
  MY/1 -> rotation EQ/2(M)
  MZ/1 -> rotation EQ/3(N)
  D/1 -> dynamics EQ/1(D)
  S/1 -> dynamics EQ/2(S)
  L/1 -> dynamics EQ/3(L)
  [p] -> dynamics EQ/4(p)
  [q] -> dynamics EQ/5(q)
  [r] -> dynamics EQ/6(r)
  thrust/1 -> dynamics EQ/7(thrust)
  [phi_eular] -> dynamics EQ/8(phi(euler angle))
  [theta_eular] -> dynamics EQ/9(theta(euler angle))
  [psi_eular] -> dynamics EQ/10(psi(euler angle))
  dynamics EQ/1(u) -> [u]
  dynamics EQ/2(v) -> [v]
  dynamics EQ/3(w) -> [w]
  [u] -> Subsystem3/1(u)
  [v] -> Subsystem3/2(v)
  [w] -> Subsystem3/3(w)
  [phi_eular] -> Subsystem3/4(phi)
  [theta_eular] -> Subsystem3/5(theta)
  [psi_eular] -> Subsystem3/6(psi)
  Subsystem3/1(alpha(H)) -> Gain1/1
  Subsystem3/2(beta(H)) -> Gain5/1
  Subsystem3/3(X(position)) -> [X_positon], X/1
  Subsystem3/4(Y(position)) -> [Y_positon], Y/1
  Subsystem3/5(Z(position)) -> [Z_positon], Z/1
  delta_s(H)/1 -> 起落架模型/1(delta_s(H))
  u_brake/1 -> 起落架模型/2(u_brake)
  rotation EQ/1(p) -> [p]
  rotation EQ/2(q) -> [q]
  rotation EQ/3(r) -> [r]
  [p] -> 姿态角/1(p)
  [q] -> 姿态角/2(q)
  [r] -> 姿态角/3(r)

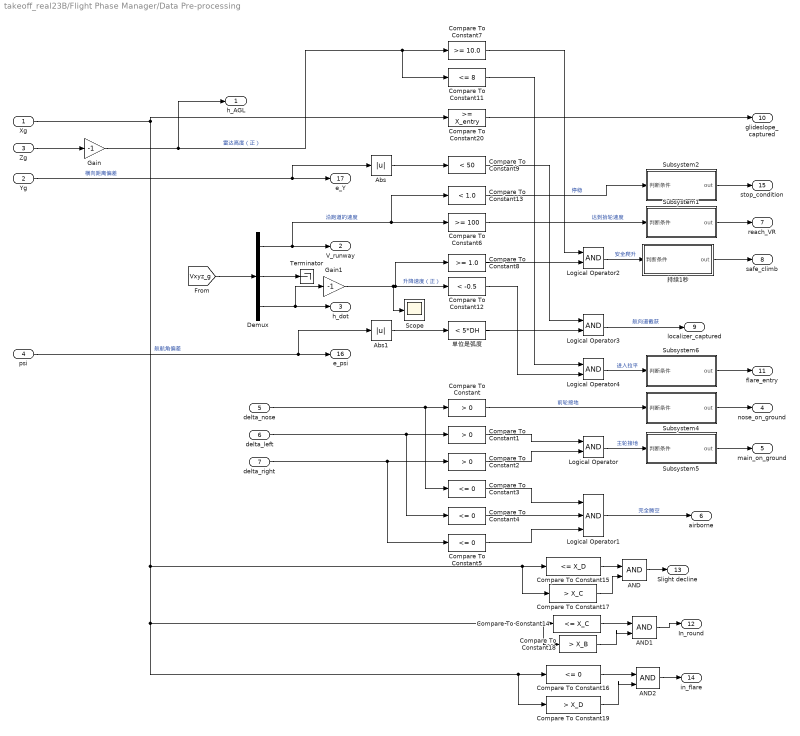
== system takeoff_real23B/Flight Phase Manager/Data Pre-processing ==
  Xg : Inport
  Yg : Inport  Port=2
  Zg : Inport  Port=3
  psi : Inport  Port=4
  delta_nose : Inport  Port=5
  delta_left : Inport  Port=6
  delta_right : Inport  Port=7
  AND : Logic  IconShape=distinctive  AllPortsSameDT=off  OutDataTypeStr=boolean
  AND1 : Logic  IconShape=distinctive  AllPortsSameDT=off  OutDataTypeStr=boolean
  AND2 : Logic  IconShape=distinctive  AllPortsSameDT=off  OutDataTypeStr=boolean
  Abs : Abs  SaturateOnIntegerOverflow=off
  Abs1 : Abs  SaturateOnIntegerOverflow=off
  Compare To Constant : simulink/Logic and Bit Operations/Compare To Constant  relop=>  const=0  OutDataTypeStr=boolean
  Compare To Constant1 : simulink/Logic and Bit Operations/Compare To Constant  relop=>  const=0  OutDataTypeStr=boolean
  Compare To Constant11 : simulink/Logic and Bit Operations/Compare To Constant  relop=<=  const=8  OutDataTypeStr=boolean
  Compare To Constant12 : simulink/Logic and Bit Operations/Compare To Constant  relop=<  const=-0.5  OutDataTypeStr=boolean
  Compare To Constant13 : simulink/Logic and Bit Operations/Compare To Constant  relop=<  const=1.0  OutDataTypeStr=boolean
  Compare To Constant14 : simulink/Logic and Bit Operations/Compare To Constant  relop=<=  const=X_C  OutDataTypeStr=boolean
  Compare To Constant15 : simulink/Logic and Bit Operations/Compare To Constant  relop=<=  const=X_D  OutDataTypeStr=boolean
  Compare To Constant{3..5,16} (4 alike) : simulink/Logic and Bit Operations/Compare To Constant  relop=<=  const=0  OutDataTypeStr=boolean
  Compare To Constant17 : simulink/Logic and Bit Operations/Compare To Constant  relop=>  const=X_C  OutDataTypeStr=boolean
  Compare To Constant18 : simulink/Logic and Bit Operations/Compare To Constant  relop=>  const=X_B  OutDataTypeStr=boolean
  Compare To Constant19 : simulink/Logic and Bit Operations/Compare To Constant  relop=>  const=X_D  OutDataTypeStr=boolean
  Compare To Constant2 : simulink/Logic and Bit Operations/Compare To Constant  relop=>  const=0  OutDataTypeStr=boolean
  Compare To Constant20 : simulink/Logic and Bit Operations/Compare To Constant  relop=>=  const=X_entry  OutDataTypeStr=boolean
  Compare To Constant6 : simulink/Logic and Bit Operations/Compare To Constant  relop=>=  const=100  OutDataTypeStr=boolean
  Compare To Constant7 : simulink/Logic and Bit Operations/Compare To Constant  relop=>=  const=10.0  OutDataTypeStr=boolean
  Compare To Constant8 : simulink/Logic and Bit Operations/Compare To Constant  relop=>=  const=1.0  OutDataTypeStr=boolean
  Compare To Constant9 : simulink/Logic and Bit Operations/Compare To Constant  relop=<  const=50  OutDataTypeStr=boolean
  Demux : Demux  Outputs=3
  Gain : Gain  Gain=-1
  Gain1 : Gain  Gain=-1
  Logical Operator{,2..4} (4 alike) : Logic  AllPortsSameDT=off  OutDataTypeStr=boolean
  Logical Operator1 : Logic  Inputs=3  AllPortsSameDT=off  OutDataTypeStr=boolean
  Scope : Scope
  Subsystem1 : Subsystem
  Subsystem2 : Subsystem
  Subsystem4 : Subsystem
  Subsystem5 : Subsystem
  Subsystem6 : Subsystem
  Terminator : Terminator
  单位是弧度 : simulink/Logic and Bit Operations/Compare To Constant  relop=<  const=5*DH  OutDataTypeStr=boolean
  持续1秒 : Subsystem
  h_AGL : Outport
  V_runway : Outport  Port=2
  h_dot : Outport  Port=3
  nose_on_ground : Outport  Port=4
  main_on_ground : Outport  Port=5
  airborne : Outport  Port=6
  reach_VR : Outport  Port=7
  safe_climb : Outport  Port=8
  localizer_captured : Outport  Port=9
  glideslope_captured : Outport  Port=10
  flare_entry : Outport  Port=11
  In_round : Outport  Port=12
  Slight decline : Outport  Port=13
  in_flare : Outport  Port=14
  stop_condition : Outport  Port=15
  e_psi : Outport  Port=16
  e_Y : Outport  Port=17
  wires:
  [Vxyz_g] -> Demux/1
  Demux/1 -> V_runway/1, Compare To Constant13/1, Compare To Constant6/1  "沿跑道的速度"
  psi/1 -> e_psi/1, Abs1/1  "航航角偏差"
  delta_nose/1 -> Compare To Constant3/1, Compare To Constant/1
  delta_left/1 -> Compare To Constant1/1, Compare To Constant4/1
  delta_right/1 -> Compare To Constant2/1, Compare To Constant5/1
  Compare To Constant1/1 -> Logical Operator/1
  Compare To Constant2/1 -> Logical Operator/2
  Compare To Constant4/1 -> Logical Operator1/2
  Compare To Constant3/1 -> Logical Operator1/1
  Compare To Constant5/1 -> Logical Operator1/3
  Compare To Constant8/1 -> Logical Operator2/2
  Compare To Constant7/1 -> Logical Operator2/1
  Abs/1 -> Compare To Constant9/1
  Abs1/1 -> 单位是弧度/1
  单位是弧度/1 -> Logical Operator3/2
  Compare To Constant9/1 -> Logical Operator3/1
  Compare To Constant11/1 -> Logical Operator4/1
  Compare To Constant12/1 -> Logical Operator4/2
  持续1秒/1(out) -> safe_climb/1
  Logical Operator3/1 -> localizer_captured/1  "航向道截获"
  Logical Operator2/1 -> 持续1秒/1(判断条件)  "安全爬升"
  Subsystem1/1(out) -> reach_VR/1
  Compare To Constant6/1 -> Subsystem1/1(判断条件)  "达到抬轮速度"
  Subsystem2/1(out) -> stop_condition/1
  Compare To Constant13/1 -> Subsystem2/1(判断条件)  "停稳"
  Logical Operator1/1 -> airborne/1  "完全腾空"
  Subsystem4/1(out) -> nose_on_ground/1
  Compare To Constant/1 -> Subsystem4/1(判断条件)  "前轮接地"
  Subsystem5/1(out) -> main_on_ground/1
  Logical Operator/1 -> Subsystem5/1(判断条件)  "主轮接地"
  Subsystem6/1(out) -> flare_entry/1
  Logical Operator4/1 -> Subsystem6/1(判断条件)  "进入拉平"
  Zg/1 -> Gain/1
  Yg/1 -> e_Y/1, Abs/1  "横向距离偏差"
  Gain1/1 -> Scope/1, Compare To Constant8/1, Compare To Constant12/1  "升降速度（正）"
  Demux/2 -> Terminator/1
  Demux/3 -> Gain1/1, h_dot/1
  Gain/1 -> Compare To Constant7/1, Compare To Constant11/1, h_AGL/1  "雷达高度（正）"
  Compare To Constant15/1 -> AND/1
  AND/1 -> Slight decline/1
  Compare To Constant17/1 -> AND/2
  AND1/1 -> In_round/1
  Compare To Constant14/1 -> AND1/1
  Compare To Constant18/1 -> AND1/2
  Compare To Constant16/1 -> AND2/1
  AND2/1 -> in_flare/1
  Compare To Constant19/1 -> AND2/2
  Xg/1 -> Compare To Constant20/1, Compare To Constant18/1, Compare To Constant14/1, Compare To Constant19/1, Compare To Constant16/1, Compare To Constant17/1, Compare To Constant15/1
  Compare To Constant20/1 -> glideslope_captured/1

== system takeoff_real23B/Guidance/1_地面制导 ==
  Flight_Phase : Inport
  e_Y : Inport  Port=2
  e_psi : Inport  Port=3
  r : Inport  Port=4
  Vxg : Inport  Port=5
  h_AGL : Inport  Port=6
  Enable : EnablePort
  Bus Creator : BusCreator  Inputs=10
  Compare To Constant : simulink/Logic and Bit Operations/Compare To Constant  relop=>=  const=11  OutDataTypeStr=boolean
  Constant1 : Constant
  Constant4 : Constant  Value=0
  Gain : Gain  Gain=-1
  Gain2 : Gain  Gain=0.08
  Gain3 : Gain  Gain=-0.85
  Gain4 : Gain  Gain=-0.2
  H_cmd : Constant  Value=-0.821594300000000
  MATLAB Function : MATLAB Function  TreatAsAtomicUnit=on  SystemSampleTime=0.001
  Sum : Sum  Inputs=|++
  Sum1 : Sum  Inputs=|++
  Switch : Switch  Criteria=u2 > Threshold  SaturateOnIntegerOverflow=off  InputSameDT=off
  Switch2 : Switch  Criteria=u2 > Threshold  SaturateOnIntegerOverflow=off  InputSameDT=off
  V_cmd1 : Constant  Value=V_flare
  ny_cmd : Constant  Value=0.0
  nz_cmd : Constant  Value=1.0
  phi_cmd : Constant  Value=0.0
  psi_cmd : Saturate  UpperLimit=25*pi/180  LowerLimit=-25*pi/180
  theta_cmd : Constant  Value=0.0
  throttle_cmd : Constant  Value=0
  Cmd_Bus : Outport
  wires:
  Flight_Phase/1 -> MATLAB Function/1(Flight_Phase), Compare To Constant/1
  nz_cmd/1 -> Bus Creator/1  "nz_cmd"
  ny_cmd/1 -> Bus Creator/2  "ny_cmd"
  phi_cmd/1 -> Bus Creator/3  "phi_cmd"
  psi_cmd/1 -> Bus Creator/4  "psi_cmd"
  theta_cmd/1 -> Bus Creator/5  "theta_cmd"
  Bus Creator/1 -> Cmd_Bus/1
  e_Y/1 -> Gain/1
  throttle_cmd/1 -> Bus Creator/7  "throttle_cmd"
  Gain/1 -> Gain2/1
  e_psi/1 -> Gain3/1
  Gain2/1 -> Sum/1
  Gain3/1 -> Sum/2
  Sum/1 -> Sum1/1
  Gain4/1 -> Sum1/2
  Sum1/1 -> psi_cmd/1
  r/1 -> Gain4/1
  MATLAB Function/1(gamma_cmd) -> Bus Creator/9  "gamma"
  H_cmd/1 -> Bus Creator/10  "H_cmd"
  Constant1/1 -> Switch/1
  V_cmd1/1 -> Switch2/3  "V_cmd"
  Switch2/1 -> Bus Creator/6  "V_cmd"
  Constant4/1 -> Switch2/1, Switch/3
  Switch/1 -> Bus Creator/8  "brake_cmd"
  Compare To Constant/1 -> Switch/2, Switch2/2
  Vxg/1 -> MATLAB Function/2(Vxg)
  h_AGL/1 -> MATLAB Function/3(h_AGL)

== system takeoff_real23B/Guidance/2_抬轮制导  ==
  Vwind_ground : Inport
  Va_safe : Inport  Port=2
  Enable : EnablePort  StatesWhenEnabling=reset
  Asin : Trigonometry  Operator=asin
  Bus Creator : BusCreator  Inputs=10
  Constant : Constant  Value=12
  Constant1 : Constant  Value=0
  Divide : Product  Inputs=*/
  Gain : Gain  Gain=DH
  Gain1 : Gain  Gain=-1
  H_cmd : Constant  Value=0
  Saturation2 : Saturate  UpperLimit=10*DH  LowerLimit=-10*DH
  Selector : Selector  InputPortWidth=3  IndexOptions=Index vector (dialog)  Indices=2  OutputSizes=1
  V_cmd : Constant  Value=200
  gamma : Constant  Value=0
  ny_cmd : Constant  Value=0
  nz_cmd : Constant
  phi_cmd : Constant  Value=0
  throttle_cmd : Constant
  cmd_Bus : Outport  InitialOutput=0
  wires:
  Constant1/1 -> Bus Creator/8  "brake_cmd"
  Saturation2/1 -> Bus Creator/4  "psi_cmd"
  V_cmd/1 -> Bus Creator/6  "V_cmd"
  throttle_cmd/1 -> Bus Creator/7  "throttle_cmd"
  nz_cmd/1 -> Bus Creator/1  "nz_cmd"
  Gain/1 -> Bus Creator/5  "theta_cmd"
  ny_cmd/1 -> Bus Creator/2  "ny_cmd"
  Bus Creator/1 -> cmd_Bus/1
  phi_cmd/1 -> Bus Creator/3  "phi_cmd"
  Constant/1 -> Gain/1
  Gain1/1 -> Saturation2/1
  Selector/1 -> Divide/1
  Divide/1 -> Asin/1
  Asin/1 -> Gain1/1
  Va_safe/1 -> Divide/2
  Vwind_ground/1 -> Selector/1
  H_cmd/1 -> Bus Creator/10  "H_cmd"
  gamma/1 -> Bus Creator/9  "gamma"

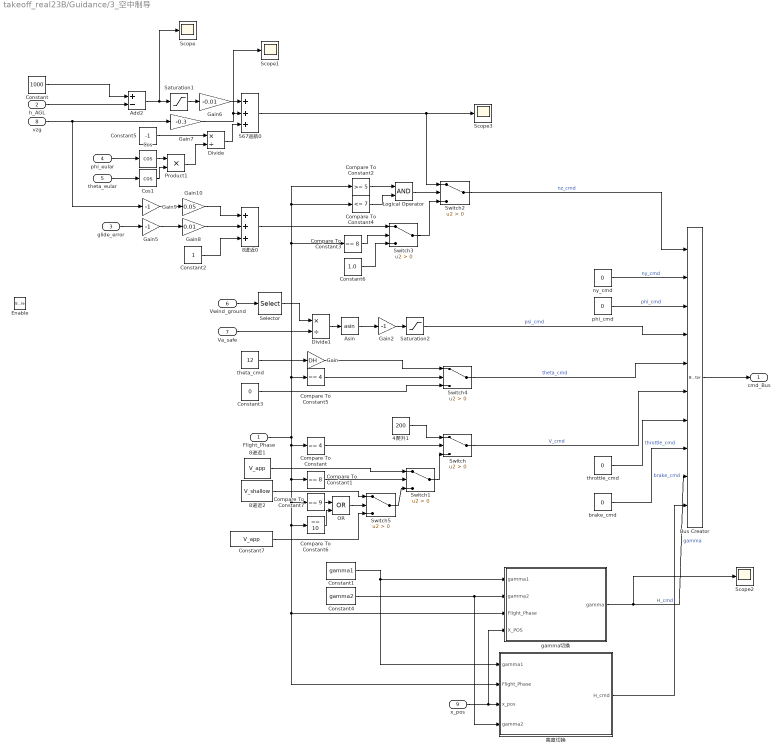
== system takeoff_real23B/Guidance/3_空中制导 ==
  Flight_Phase : Inport
  h_AGL : Inport  Port=2
  glide_error : Inport  Port=3
  phi_eular : Inport  Port=4
  theta_eular : Inport  Port=5
  Vwind_ground : Inport  Port=6
  Va_safe : Inport  Port=7
  vzg : Inport  Port=8
  x_pos : Inport  Port=9
  Enable : EnablePort
  4爬升1 : Constant  Value=200
  567巡航0 : Sum  Inputs=+++
  8进近0 : Sum  Inputs=+++
  8进近1 : Constant  Value=V_app
  8进近2 : Constant  Value=V_shallow
  Add2 : Sum  Inputs=+-
  Asin : Trigonometry  Operator=asin
  Bus Creator : BusCreator  Inputs=10
  Compare To Constant : simulink/Logic and Bit Operations/Compare To Constant  relop===  const=4  OutDataTypeStr=boolean
  Compare To Constant1 : simulink/Logic and Bit Operations/Compare To Constant  relop===  const=8  OutDataTypeStr=boolean
  Compare To Constant2 : simulink/Logic and Bit Operations/Compare To Constant  relop=>=  const=5  OutDataTypeStr=boolean
  Compare To Constant3 : simulink/Logic and Bit Operations/Compare To Constant  relop===  const=8  OutDataTypeStr=boolean
  Compare To Constant4 : simulink/Logic and Bit Operations/Compare To Constant  relop=<=  const=7  OutDataTypeStr=boolean
  Compare To Constant5 : simulink/Logic and Bit Operations/Compare To Constant  relop===  const=4  OutDataTypeStr=boolean
  Compare To Constant6 : simulink/Logic and Bit Operations/Compare To Constant  relop===  const=10  OutDataTypeStr=boolean
  Compare To Constant7 : simulink/Logic and Bit Operations/Compare To Constant  relop===  const=9  OutDataTypeStr=boolean
  Constant : Constant  Value=1000
  Constant1 : Constant  Value=gamma1
  Constant2 : Constant
  Constant3 : Constant  Value=0
  Constant4 : Constant  Value=gamma2
  Constant5 : Constant  Value=-1
  Constant6 : Constant  Value=1.0
  Constant7 : Constant  Value=V_app
  Cos : Trigonometry  Operator=cos
  Cos1 : Trigonometry  Operator=cos
  Divide : Product  Inputs=*/
  Divide1 : Product  Inputs=*/
  Gain : Gain  Gain=DH
  Gain10 : Gain  Gain=0.05
  Gain2 : Gain  Gain=-1
  Gain5 : Gain  Gain=-1
  Gain6 : Gain  Gain=-0.01
  Gain7 : Gain  Gain=-0.3
  Gain8 : Gain  Gain=0.01
  Gain9 : Gain  Gain=-1
  Logical Operator : Logic  AllPortsSameDT=off  OutDataTypeStr=boolean
  OR : Logic  Operator=OR  IconShape=distinctive  AllPortsSameDT=off  OutDataTypeStr=boolean
  Product1 : Product
  Saturation1 : Saturate  UpperLimit=100  LowerLimit=-100
  Saturation2 : Saturate  UpperLimit=10*DH  LowerLimit=-10*DH
  Scope{,1..3} (4 alike) : Scope
  Selector : Selector  InputPortWidth=3  IndexOptions=Index vector (dialog)  Indices=2  OutputSizes=1
  Switch{,1..5} (6 alike) : Switch  Criteria=u2 > Threshold  SaturateOnIntegerOverflow=off  InputSameDT=off
  brake_cmd : Constant  Value=0
  gamma切换 : Subsystem
  ny_cmd : Constant  Value=0
  phi_cmd : Constant  Value=0
  theta_cmd : Constant  Value=12
  throttle_cmd : Constant  Value=0
  高度切换 : Subsystem
  cmd_Bus : Outport
  wires:
  brake_cmd/1 -> Bus Creator/8  "brake_cmd"
  Saturation2/1 -> Bus Creator/4  "psi_cmd"
  Switch/1 -> Bus Creator/6  "V_cmd"
  Bus Creator/1 -> cmd_Bus/1
  Compare To Constant/1 -> Switch/2
  4爬升1/1 -> Switch/1
  Switch1/1 -> Switch/3
  Compare To Constant1/1 -> Switch1/2
  8进近1/1 -> Switch1/1
  vzg/1 -> Gain9/1, Gain7/1
  Gain6/1 -> 567巡航0/1
  Gain7/1 -> Scope1/1, 567巡航0/2
  h_AGL/1 -> Add2/2
  Constant/1 -> Add2/1
  glide_error/1 -> Gain5/1
  Gain5/1 -> Gain8/1
  Gain8/1 -> 8进近0/2
  Gain9/1 -> Gain10/1
  Gain10/1 -> 8进近0/1
  Constant2/1 -> 8进近0/3
  Compare To Constant3/1 -> Switch3/2
  Flight_Phase/1 -> Compare To Constant6/1, 高度切换/2(Flight_Phase), gamma切换/3(Flight_Phase), Compare To Constant7/1, Compare To Constant1/1, Compare To Constant/1, Compare To Constant2/1, Compare To Constant4/1, Compare To Constant3/1, Compare To Constant5/1
  throttle_cmd/1 -> Bus Creator/7  "throttle_cmd"
  Compare To Constant2/1 -> Logical Operator/1
  Compare To Constant4/1 -> Logical Operator/2
  Logical Operator/1 -> Switch2/2
  567巡航0/1 -> Scope3/1, Switch2/1
  Switch3/1 -> Switch2/3
  Constant6/1 -> Switch3/3
  8进近0/1 -> Switch3/1
  Switch2/1 -> Bus Creator/1  "nz_cmd"
  Compare To Constant5/1 -> Switch4/2
  Switch4/1 -> Bus Creator/5  "theta_cmd"
  Constant3/1 -> Switch4/3
  theta_cmd/1 -> Gain/1
  phi_eular/1 -> Cos/1
  Cos/1 -> Product1/1
  Divide/1 -> 567巡航0/3
  Constant5/1 -> Divide/1
  Product1/1 -> Divide/2
  Cos1/1 -> Product1/2
  Asin/1 -> Gain2/1
  Gain2/1 -> Saturation2/1
  Divide1/1 -> Asin/1
  Selector/1 -> Divide1/1
  Va_safe/1 -> Divide1/2
  ny_cmd/1 -> Bus Creator/2  "ny_cmd"
  phi_cmd/1 -> Bus Creator/3  "phi_cmd"
  Gain/1 -> Switch4/1
  theta_eular/1 -> Cos1/1
  Vwind_ground/1 -> Selector/1
  Saturation1/1 -> Gain6/1
  Add2/1 -> Scope/1, Saturation1/1
  Constant1/1 -> 高度切换/1(gamma1), gamma切换/1(gamma1)
  gamma切换/1(gamma) -> Scope2/1, Bus Creator/9  "gamma"
  Constant4/1 -> 高度切换/4(gamma2), gamma切换/2(gamma2)
  x_pos/1 -> gamma切换/4(X_POS), 高度切换/3(x_pos)
  高度切换/1(H_cmd) -> Bus Creator/10  "H_cmd"
  Compare To Constant7/1 -> OR/1
  Compare To Constant6/1 -> OR/2
  OR/1 -> Switch5/2
  Switch5/1 -> Switch1/3
  8进近2/1 -> Switch5/1
  Constant7/1 -> Switch5/3

== system takeoff_real23B/Guidance/4_拉平制导 ==
  e_Z : Inport
  e_psi : Inport  Port=2
  X_pos : Inport  Port=3
  Flight_Phase : Inport  Port=4
  Vxg : Inport  Port=5
  Enable : EnablePort
  Add3 : Sum  Inputs=+-
  Bus Creator : BusCreator  Inputs=10
  Constant1 : Constant
  Constant2 : Constant  Value=0
  Constant3 : Constant  Value=0
  Constant4 : Constant  Value=0
  Gain2 : Gain  Gain=-1
  Gain3 : Gain  Gain=-1
  Gain4 : Gain  Gain=0.02
  Gain5 : Gain  Gain=0.5
  MATLAB Function : MATLAB Function  TreatAsAtomicUnit=on
  MATLAB Function1 : MATLAB Function  TreatAsAtomicUnit=on  SystemSampleTime=0.001
  Saturation1 : Saturate  UpperLimit=0.17  LowerLimit=-0.17
  Scope : Scope
  V_cmd : Constant  Value=V_flare
  theta_cmd : Constant  Value=0
  throttle_cmd : Constant  Value=0
  cmd_Bus : Outport
  wires:
  Saturation1/1 -> Bus Creator/4  "psi_cmd"
  V_cmd/1 -> Bus Creator/6  "V_cmd"
  throttle_cmd/1 -> Bus Creator/7  "throttle_cmd"
  theta_cmd/1 -> Bus Creator/5  "theta_cmd"
  Constant3/1 -> Bus Creator/2  "ny_cmd"
  Bus Creator/1 -> cmd_Bus/1
  Constant2/1 -> Bus Creator/3  "phi_cmd"
  e_Z/1 -> Gain2/1
  e_psi/1 -> Gain3/1
  Gain2/1 -> Gain4/1
  Gain3/1 -> Gain5/1
  Gain4/1 -> Add3/1
  Gain5/1 -> Add3/2
  Add3/1 -> Saturation1/1
  X_pos/1 -> MATLAB Function1/3(X_pos), MATLAB Function/1(X_pos)
  Constant1/1 -> Bus Creator/1  "nz_cmd"
  MATLAB Function1/1(gamma_cmd) -> Bus Creator/9  "gamma"
  MATLAB Function/1(H_cmd) -> Bus Creator/10  "H_cmd"
  Flight_Phase/1 -> MATLAB Function1/1(Flight_Phase)
  Vxg/1 -> MATLAB Function1/2(Vxg)
  Constant4/1 -> Bus Creator/8  "brake_cmd"

== system takeoff_real23B/controller1/1_Pitch_Ctrl ==
  Flight_Phase : Inport
  nz_cmd : Inport  Port=2
  theta_cmd : Inport  Port=3
  nz : Inport  Port=4
  theta : Inport  Port=5
  q : Inport  Port=6
  H_cmd : Inport  Port=7
  gamma : Inport  Port=8
  234俯仰角控制 : Subsystem
  567三回路控制 : Subsystem
  89101112_着陆俯仰控制 : Subsystem
  Clock_blend : Clock
  Compare To Constant1 : simulink/Logic and Bit Operations/Compare To Constant  relop=>=  const=5  OutDataTypeStr=boolean
  Compare To Constant4 : simulink/Logic and Bit Operations/Compare To Constant  relop=<=  const=7  OutDataTypeStr=boolean
  Compare To Constant6 : simulink/Logic and Bit Operations/Compare To Constant  relop=>=  const=5  OutDataTypeStr=boolean
  Compare To Constant7 : simulink/Logic and Bit Operations/Compare To Constant  relop=<=  const=7  OutDataTypeStr=boolean
  Compare To Constant9 : simulink/Logic and Bit Operations/Compare To Constant  relop=<  const=5  OutDataTypeStr=boolean
  Gain3 : Gain  Gain=180/pi
  Logical Operator2 : Logic  Operator=NOT  AllPortsSameDT=off  OutDataTypeStr=boolean
  Logical Operator3 : Logic  Operator=OR  AllPortsSameDT=off  OutDataTypeStr=boolean
  Logical Operator4 : Logic  Operator=OR  AllPortsSameDT=off  OutDataTypeStr=boolean
  Pitch45Blend : MATLAB Function  TreatAsAtomicUnit=on  SystemSampleTime=0.001
  Saturation : Saturate  UpperLimit=25  LowerLimit=-25
  Scope1 : Scope
  Scope2 : Scope
  Scope3 : Scope
  Switch : Switch  Criteria=u2 > Threshold  SaturateOnIntegerOverflow=off  InputSameDT=off
  Switch1 : Switch  Criteria=u2 > Threshold  SaturateOnIntegerOverflow=off  InputSameDT=off
  T_blend : Constant  Value=5
  de_cmd : Outport
  wires:
  Pitch45Blend/1(de_cmd_rad) -> Gain3/1
  Flight_Phase/1 -> Compare To Constant6/1, Compare To Constant1/1, Compare To Constant4/1, Compare To Constant7/1, Compare To Constant9/1
  Pitch45Blend/2(lambda) -> Scope1/1
  Gain3/1 -> Saturation/1
  theta_cmd/1 -> 234俯仰角控制/1(theta_cmd)
  theta/1 -> 234俯仰角控制/2(theta)
  nz_cmd/1 -> 567三回路控制/1(nz_cmd)
  nz/1 -> 567三回路控制/2(nz)
  q/1 -> 567三回路控制/3(q), 234俯仰角控制/3(q)
  Logical Operator2/1 -> 567三回路控制/4(复位)
  567三回路控制/1(de_nz_rad) -> Scope3/1, Switch/1
  Compare To Constant1/1 -> Logical Operator3/2
  Compare To Constant4/1 -> Logical Operator3/1
  Logical Operator3/1 -> Switch/2
  Switch/1 -> Switch1/3
  89101112_着陆俯仰控制/1(de) -> Switch/3
  [Vg] -> 89101112_着陆俯仰控制/1(Vg)
  H_cmd/1 -> 89101112_着陆俯仰控制/3(h_cmd)
  gamma/1 -> 89101112_着陆俯仰控制/2(gamma)
  Switch1/1 -> Scope2/1, de_cmd/1
  Compare To Constant6/1 -> Logical Operator4/2
  Compare To Constant7/1 -> Logical Operator4/1
  Logical Operator4/1 -> Logical Operator2/1
  234俯仰角控制/1(de_theta_rad) -> Switch1/1
  Compare To Constant9/1 -> Switch1/2
